simulink model "Modal_Control_Closed_Disturp_Integ"  (R2018b)
settings: Solver=VariableStepAuto  StartTime=0.0  StopTime=200  RelTol=1e-3
values from neighbouring files (symbols this model uses):
  alpha = 0.5736    [constants.m]
  c_damp = 0.00495    [constants.m]
  delay = 0.8    [constants.m]
  dis_torque = 0.001    [constants.m]
  in_nu = 0.0001    [constants.m]
  J_r = 0.0004    [constants.m]
  J_s = 31.38    [constants.m]
  Kint = real(W/(sys.c*V))    [Micro_Sat_Closed_Loop.m]
  noise = 10^-9    (= 1e-09)    [constants.m]
  T_sat = 0.05    [constants.m]
  time_cons = 0.5    [constants.m]
  w_mode = 2.6268    [constants.m]
  w_sat = 2800*2*pi/60    (= 293.215314335)    [constants.m]
settings Model: Creator=Yavuz  LastModifiedBy=Yavuz
settings DebuggingCC: AlgebraicLoopMsg=none

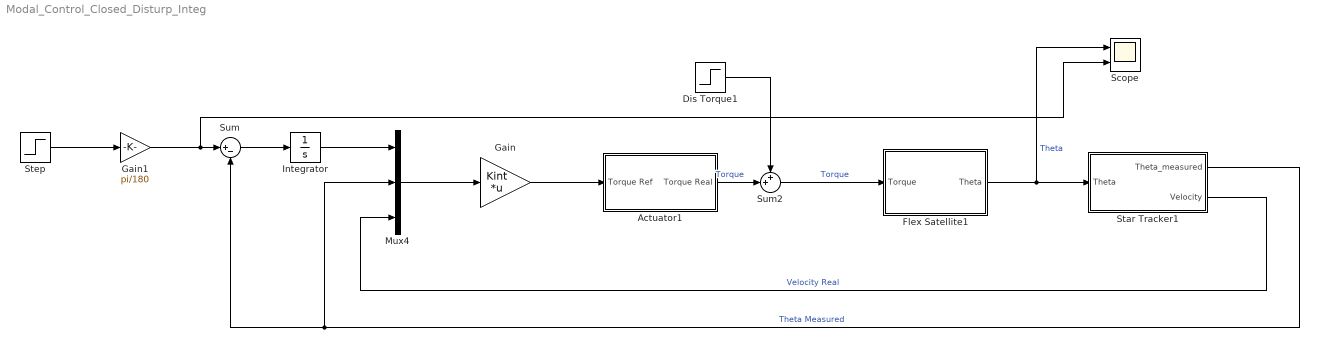
== system Modal_Control_Closed_Disturp_Integ ==
  Actuator1 : Subsystem
  Dis Torque1 : Step  Time=100  After=dis_torque  SampleTime=0
  Flex Satellite1 : Subsystem
  Gain : Gain  Gain=Kint  Multiplication=Matrix(K*u)
  Gain1 : Gain  Gain=pi/180
  Integrator : Integrator
  Mux4 : Mux  Inputs=3
  Scope : Scope  NumInputPorts=2
  Star Tracker1 : Subsystem
  Step : Step  Time=0  After=2.5  SampleTime=0
  Sum : Sum  Inputs=|+-
  Sum2 : Sum  Inputs=++|
  wires:
  Step/1 -> Gain1/1
  Sum/1 -> Integrator/1
  Integrator/1 -> Mux4/1
  Mux4/1 -> Gain/1
  Actuator1/1(Torque Real) -> Sum2/2  "Torque"
  Dis Torque1/1 -> Sum2/1
  Gain/1 -> Actuator1/1(Torque Ref)
  Sum2/1 -> Flex Satellite1/1(Torque)  "Torque"
  Flex Satellite1/1(Theta) -> Scope/1, Star Tracker1/1(Theta)  "Theta"
  Star Tracker1/1(Theta_measured) -> Sum/2, Mux4/2  "Theta Measured"
  Star Tracker1/2(Velocity) -> Mux4/3  "Velocity Real"
  Gain1/1 -> Sum/1, Scope/2

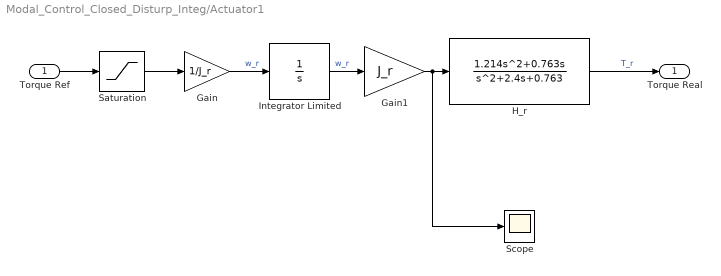
== system Modal_Control_Closed_Disturp_Integ/Actuator1 ==
  Torque Ref : Inport
  Gain : Gain  Gain=1/J_r
  Gain1 : Gain  Gain=J_r
  H_r : TransferFcn  Numerator=[1.214 0.763 0]  Denominator=[1 2.4 0.763]
  Integrator Limited : Integrator  LimitOutput=on  UpperSaturationLimit=w_sat  LowerSaturationLimit=-w_sat
  Saturation : Saturate  UpperLimit=T_sat  LowerLimit=-T_sat
  Scope : Scope
  Torque Real : Outport
  wires:
  Gain1/1 -> Scope/1, H_r/1
  H_r/1 -> Torque Real/1  "T_r"
  Saturation/1 -> Gain/1
  Torque Ref/1 -> Saturation/1
  Gain/1 -> Integrator Limited/1  "w_r"
  Integrator Limited/1 -> Gain1/1  "w_r"

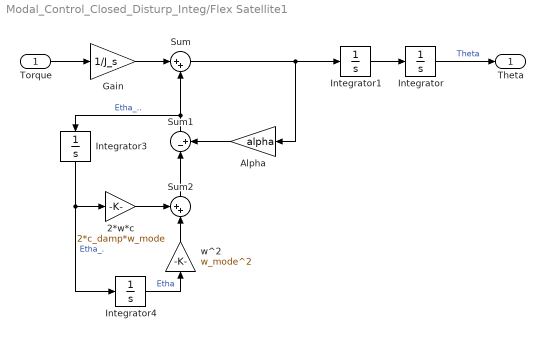
== system Modal_Control_Closed_Disturp_Integ/Flex Satellite1 ==
  Torque : Inport
  2*w*c : Gain  Gain=2*c_damp*w_mode
  Alpha : Gain  Gain=alpha
  Gain : Gain  Gain=1/J_s
  Integrator : Integrator
  Integrator1 : Integrator
  Integrator3 : Integrator
  Integrator4 : Integrator  InitialCondition=in_nu
  Sum : Sum  Inputs=|++
  Sum1 : Sum  Inputs=|-+
  Sum2 : Sum  Inputs=++|
  w^2 : Gain  Gain=w_mode^2
  Theta : Outport
  wires:
  Sum/1 -> Integrator1/1, Alpha/1
  Sum1/1 -> Integrator3/1, Sum/2  "Etha_.."
  Gain/1 -> Sum/1
  Integrator1/1 -> Integrator/1
  Integrator3/1 -> Integrator4/1, 2*w*c/1  "Etha_."
  Sum2/1 -> Sum1/1
  Torque/1 -> Gain/1
  2*w*c/1 -> Sum2/1
  Integrator/1 -> Theta/1  "Theta"
  w^2/1 -> Sum2/2
  Integrator4/1 -> w^2/1  "Etha"
  Alpha/1 -> Sum1/2

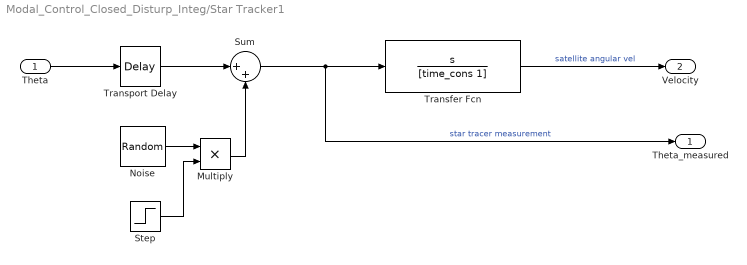
== system Modal_Control_Closed_Disturp_Integ/Star Tracker1 ==
  Theta : Inport
  Multiply : Product
  Noise : RandomNumber  Variance=noise  SampleTime=0.1
  Step : Step  Time=160  SampleTime=0
  Sum : Sum  Inputs=|++
  Transfer Fcn : TransferFcn  Numerator=[1 0]  Denominator=[time_cons 1]
  Transport Delay : TransportDelay  DelayTime=delay
  Theta_measured : Outport
  Velocity : Outport  Port=2
  wires:
  Sum/1 -> Theta_measured/1, Transfer Fcn/1  "star tracer measurement"
  Transfer Fcn/1 -> Velocity/1  "satellite angular vel"
  Multiply/1 -> Sum/2
  Noise/1 -> Multiply/1
  Theta/1 -> Transport Delay/1
  Step/1 -> Multiply/2
  Transport Delay/1 -> Sum/1
